simulink model "V40AeroDynamics_edit_3D"  (R2017b)
settings: Solver=VariableStepAuto  StartTime=0.0  StopTime=500  RelTol=1e-3
values from neighbouring files (symbols this model uses):
  A = [ 0        0        0        1 ... (first row only)    [LinearV40.m]
  B = [ 0         0 ... (first row only)    [LinearV40.m]
  b_ref = 5.1    [V40_CFD.mat]
  C = [1       0       0       0 ... (first row only)    [LinearV40.m]
  c_bar = 0.321    [V40_CFD.mat]
  CG_ref_x = 1.38    [V40_CFD.mat]
  CG_ref_z = 0    [V40_CFD.mat]
  CL0 = 0.3831    [V40_CFD.mat]
  Clp = -0.595    [V40_CFD.mat]
  Clr = 0.005    [V40_CFD.mat]
  Cm0 = 0.109    [V40_CFD.mat]
  Cmq = -24.09    [V40_CFD.mat]
  Cnp = 0    [V40_CFD.mat]
  Cnr = -0.023    [V40_CFD.mat]
  CX_d_ca_l =     [V40_CFD.mat]
  CX_d_ca_r =     [V40_CFD.mat]
  CX_d_ea_l =     [V40_CFD.mat]
  CX_d_ea_r =     [V40_CFD.mat]
  CX_d_r =     [V40_CFD.mat]
  D = zeros(size(C,1),2)    [LinearV40.m]
  D_CL_alpha = [-1.0711 -0.8677 -0.6557 -0.4384 -0.2189 0 0.2148 0.422 0.6186 0.8018 0.9688 1.1173 ... (17 elements, 1x17)]    [V40_CFD.mat]
  D_Cm_alpha = [0.0153 0.0193 0.0198 0.0168 0.0102 0 -0.0133 -0.0293 -0.0475 -0.0672 -0.0875 -0.1073 ... (17 elements, 1x17)]    [V40_CFD.mat]
  DCD_alpha = [0.1342 0.0942 0.065 0.0469 0.0395 0.0429 0.0567 0.0807 0.1143 0.1571 0.2086 0.2683 ... (17 elements, 1x17)]    [V40_CFD.mat]
  DCX_beta =     [V40_CFD.mat]
  g = 9.79    [trim_v40.m]    (also in trim_v40_3D.m = 9.8)
  Iv = [13.1154, 0, 0; 0, 9.9543, 0; 0, 0, 15.7149]    [trim_v40.m]    (also in trim_v40_3D.m)
  pitchTheta0 = 0.0521    [LinearV40.m]
  q0 = 0    [LinearV40.m]    (also in trim_v40.m; trim_v40_3D.m)
  rho = 1.213    [trim_v40.m]    (also in trim_v40_3D.m)
  S_ref = 1.4    [V40_CFD.mat]
  Thrust = 39.9    [LinearV40.m]    (also in trim_v40_3D.m = 64.7)
  u0 = 26.152    [LinearV40.m]    (also in trim_v40.m = Vg(1); trim_v40_3D.m = Vg(1))
  w0 = 1.231    [LinearV40.m]    (also in trim_v40.m = Vg(3); trim_v40_3D.m = Vg(3))
  x0 = 0    [LinearV40.m]    (also in trim_v40.m; trim_v40_3D.m)
  x_CG = 1.38-0.043    (= 1.337)    [trim_v40.m]    (also in trim_v40_3D.m)
  z0 = -200    [LinearV40.m]    (also in trim_v40.m; trim_v40_3D.m)
  z_CG = 0    [trim_v40.m]    (also in trim_v40_3D.m)
libraries: simulink_extras x3, shared3dof x1, aerolibasang x1, aerolibtransform2 x1
(part 2 of 2)

== system V40AeroDynamics_edit_3D/Forces & Moments/summation/coef computation3 ==
  In : Inport
  Add1 : Sum  Inputs=++++++++
  Demux : Demux  Outputs=8
  Out : Outport
  wires:
  In/1 -> Demux/1
  Add1/1 -> Out/1
  Demux/7 -> Add1/7
  Demux/1 -> Add1/1
  Demux/2 -> Add1/2
  Demux/3 -> Add1/3
  Demux/4 -> Add1/4
  Demux/5 -> Add1/5
  Demux/6 -> Add1/6
  Demux/8 -> Add1/8

== system V40AeroDynamics_edit_3D/Forces & Moments/summation/coef computation4 ==
  In : Inport
  Add1 : Sum  Inputs=++++++++++
  Demux : Demux  Outputs=10
  Out : Outport
  wires:
  Add1/1 -> Out/1
  In/1 -> Demux/1
  Demux/1 -> Add1/1
  Demux/2 -> Add1/2
  Demux/3 -> Add1/3
  Demux/4 -> Add1/4
  Demux/5 -> Add1/5
  Demux/6 -> Add1/6
  Demux/7 -> Add1/7
  Demux/8 -> Add1/8
  Demux/9 -> Add1/9
  Demux/10 -> Add1/10

== system V40AeroDynamics_edit_3D/Forces & Moments/summation/coef computation5 ==
  In : Inport
  Add1 : Sum  Inputs=++++++++
  Demux : Demux  Outputs=8
  Out : Outport
  wires:
  Add1/1 -> Out/1
  In/1 -> Demux/1
  Demux/1 -> Add1/1
  Demux/2 -> Add1/2
  Demux/3 -> Add1/3
  Demux/4 -> Add1/4
  Demux/5 -> Add1/5
  Demux/6 -> Add1/6
  Demux/7 -> Add1/7
  Demux/8 -> Add1/8
